simulink model "Geneva_Drive"  (R2014b)
settings: Solver=ode15s  StartTime=0.0  StopTime=30  MaxStep=1e-2  RelTol=1e-4  AbsTol=1e-5
PostLoadFcn:
  | set_param(bdroot,'IgnoredZcDiagnostic','none')
  | warning off sm:compiler:topologyAnalysis:DanglingBlock
StartFcn:
  | tic;
StopFcn:
  | Elapsed_Sim_Time = toc;
  | disp(['Elapsed Sim Time = ' num2str(Elapsed_Sim_Time)]);
undefined symbols (not defined in the file): X, Y, Z
libraries: sm_lib x44, Contact_Forces_Lib x20, nesl_utility x5, simulink x1
(part 2 of 2)

== system Geneva_Drive/Contact Forces/Drive Pin to G Slots/Sensing1 ==
  S : Inport
  Bus Selector : BusSelector  OutputSignals=FCir.Fx,FCir.Fy  OutputAsBus=on
  tag scope: Frc_GLine2=global
  wires:
  S/1 -> Bus Selector/1
  Bus Selector/1 -> [Frc_GLine2]

== system Geneva_Drive/Contact Forces/Drive Pin to G Slots/Sensing2 ==
  S : Inport
  Bus Selector : BusSelector  OutputSignals=FCir.Fx,FCir.Fy  OutputAsBus=on
  tag scope: Frc_GLine3=global
  wires:
  S/1 -> Bus Selector/1
  Bus Selector/1 -> [Frc_GLine3]

== system Geneva_Drive/Contact Forces/Drive Pin to G Slots/Sensing3 ==
  S : Inport
  Bus Selector : BusSelector  OutputSignals=FCir.Fx,FCir.Fy  OutputAsBus=on
  tag scope: Frc_GLine1=global
  wires:
  S/1 -> Bus Selector/1
  Bus Selector/1 -> [Frc_GLine1]

== system Geneva_Drive/Contact Forces/Drive Pin to G Slots/Sensing4 ==
  S : Inport
  Bus Selector : BusSelector  OutputSignals=FCir.Fx,FCir.Fy  OutputAsBus=on
  tag scope: Frc_GLine4=global
  wires:
  S/1 -> Bus Selector/1
  Bus Selector/1 -> [Frc_GLine4]

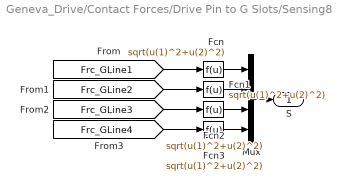
== system Geneva_Drive/Contact Forces/Drive Pin to G Slots/Sensing8 ==
  Fcn{,1..3} (4 alike) : Fcn  Expr=sqrt(u(1)^2+u(2)^2)
  Mux : Mux
  S : Outport
  wires:
  Fcn3/1 -> Mux/4
  Fcn2/1 -> Mux/3
  Fcn1/1 -> Mux/2
  Fcn/1 -> Mux/1
  [Frc_GLine4] -> Fcn3/1
  [Frc_GLine2] -> Fcn1/1
  [Frc_GLine3] -> Fcn2/1
  [Frc_GLine1] -> Fcn/1
  Mux/1 -> S/1

== system Geneva_Drive/Contact Forces/Drive Shl to G Arc/Sensing ==
  S : Inport
  Bus Selector : BusSelector  OutputSignals=Normal Force
  tag scope: Frc_A2SA=global
  wires:
  S/1 -> Bus Selector/1
  Bus Selector/1 -> [Frc_A2SA]  "<Normal Force>"

== system Geneva_Drive/Contact Forces/Drive Shl to G Arc/Sensing1 ==
  S : Inport
  Bus Selector : BusSelector  OutputSignals=Normal Force
  tag scope: Frc_A2SB=global
  wires:
  S/1 -> Bus Selector/1
  Bus Selector/1 -> [Frc_A2SB]  "<Normal Force>"

== system Geneva_Drive/Contact Forces/Drive Shl to G Arc/Sensing2 ==
  S : Inport
  Bus Selector : BusSelector  OutputSignals=Normal Force
  tag scope: Frc_A3SA=global
  wires:
  S/1 -> Bus Selector/1
  Bus Selector/1 -> [Frc_A3SA]  "<Normal Force>"

== system Geneva_Drive/Contact Forces/Drive Shl to G Arc/Sensing3 ==
  S : Inport
  Bus Selector : BusSelector  OutputSignals=Normal Force
  tag scope: Frc_A3SB=global
  wires:
  S/1 -> Bus Selector/1
  Bus Selector/1 -> [Frc_A3SB]  "<Normal Force>"

== system Geneva_Drive/Contact Forces/Drive Shl to G Arc/Sensing4 ==
  S : Inport
  Bus Selector : BusSelector  OutputSignals=Normal Force
  tag scope: Frc_A4SA=global
  wires:
  S/1 -> Bus Selector/1
  Bus Selector/1 -> [Frc_A4SA]  "<Normal Force>"

== system Geneva_Drive/Contact Forces/Drive Shl to G Arc/Sensing5 ==
  S : Inport
  Bus Selector : BusSelector  OutputSignals=Normal Force
  tag scope: Frc_A4SB=global
  wires:
  S/1 -> Bus Selector/1
  Bus Selector/1 -> [Frc_A4SB]  "<Normal Force>"

== system Geneva_Drive/Contact Forces/Drive Shl to G Arc/Sensing6 ==
  S : Inport
  Bus Selector : BusSelector  OutputSignals=Normal Force
  tag scope: Frc_A1SA=global
  wires:
  S/1 -> Bus Selector/1
  Bus Selector/1 -> [Frc_A1SA]  "<Normal Force>"

== system Geneva_Drive/Contact Forces/Drive Shl to G Arc/Sensing7 ==
  S : Inport
  Bus Selector : BusSelector  OutputSignals=Normal Force
  tag scope: Frc_A1SB=global
  wires:
  S/1 -> Bus Selector/1
  Bus Selector/1 -> [Frc_A1SB]  "<Normal Force>"

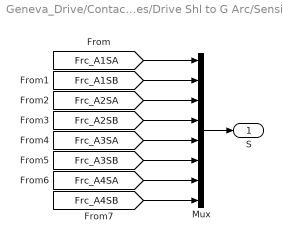
== system Geneva_Drive/Contact Forces/Drive Shl to G Arc/Sensing8 ==
  Mux : Mux  Inputs=8
  S : Outport
  wires:
  [Frc_A3SB] -> Mux/6
  [Frc_A3SA] -> Mux/5
  [Frc_A4SB] -> Mux/8
  [Frc_A4SA] -> Mux/7
  [Frc_A2SB] -> Mux/4
  [Frc_A1SB] -> Mux/2
  [Frc_A2SA] -> Mux/3
  [Frc_A1SA] -> Mux/1
  Mux/1 -> S/1

== system Geneva_Drive/Contact Forces/Drive Shl to G Tip/Sensing ==
  S : Inport
  Bus Selector : BusSelector  OutputSignals=Normal Force
  tag scope: Frc_gt2=global
  wires:
  S/1 -> Bus Selector/1
  Bus Selector/1 -> [Frc_gt2]  "<Normal Force>"

== system Geneva_Drive/Contact Forces/Drive Shl to G Tip/Sensing1 ==
  S : Inport
  Bus Selector : BusSelector  OutputSignals=Normal Force
  tag scope: Frc_gt7=global
  wires:
  S/1 -> Bus Selector/1
  Bus Selector/1 -> [Frc_gt7]  "<Normal Force>"

== system Geneva_Drive/Contact Forces/Drive Shl to G Tip/Sensing2 ==
  S : Inport
  Bus Selector : BusSelector  OutputSignals=Normal Force
  tag scope: Frc_gt6=global
  wires:
  S/1 -> Bus Selector/1
  Bus Selector/1 -> [Frc_gt6]  "<Normal Force>"

== system Geneva_Drive/Contact Forces/Drive Shl to G Tip/Sensing3 ==
  S : Inport
  Bus Selector : BusSelector  OutputSignals=Normal Force
  tag scope: Frc_gt3=global
  wires:
  S/1 -> Bus Selector/1
  Bus Selector/1 -> [Frc_gt3]  "<Normal Force>"

== system Geneva_Drive/Contact Forces/Drive Shl to G Tip/Sensing4 ==
  S : Inport
  Bus Selector : BusSelector  OutputSignals=Normal Force
  tag scope: Frc_gt4=global
  wires:
  S/1 -> Bus Selector/1
  Bus Selector/1 -> [Frc_gt4]  "<Normal Force>"

== system Geneva_Drive/Contact Forces/Drive Shl to G Tip/Sensing5 ==
  S : Inport
  Bus Selector : BusSelector  OutputSignals=Normal Force
  tag scope: Frc_gt1=global
  wires:
  S/1 -> Bus Selector/1
  Bus Selector/1 -> [Frc_gt1]  "<Normal Force>"

== system Geneva_Drive/Contact Forces/Drive Shl to G Tip/Sensing6 ==
  S : Inport
  Bus Selector : BusSelector  OutputSignals=Normal Force
  tag scope: Frc_gt8=global
  wires:
  S/1 -> Bus Selector/1
  Bus Selector/1 -> [Frc_gt8]  "<Normal Force>"

== system Geneva_Drive/Contact Forces/Drive Shl to G Tip/Sensing7 ==
  S : Inport
  Bus Selector : BusSelector  OutputSignals=Normal Force
  tag scope: Frc_gt5=global
  wires:
  S/1 -> Bus Selector/1
  Bus Selector/1 -> [Frc_gt5]  "<Normal Force>"

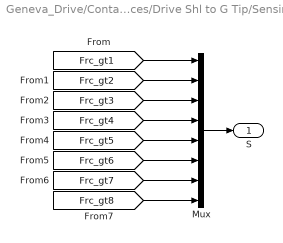
== system Geneva_Drive/Contact Forces/Drive Shl to G Tip/Sensing8 ==
  Mux : Mux  Inputs=8
  S : Outport
  wires:
  [Frc_gt6] -> Mux/6
  [Frc_gt5] -> Mux/5
  [Frc_gt8] -> Mux/8
  [Frc_gt7] -> Mux/7
  [Frc_gt4] -> Mux/4
  [Frc_gt2] -> Mux/2
  [Frc_gt3] -> Mux/3
  [Frc_gt1] -> Mux/1
  Mux/1 -> S/1
